simulink model "discrete_error_state_kalman"  (R2016a)
settings: Solver=VariableStepAuto  StartTime=0.0  StopTime=10.0  RelTol=1e-3
settings Model: Creator=mgreiff  LastModifiedBy=mgreiff
settings DataIOCC: LimitDataPoints=on
settings DebuggingCC: AllowSymbolicDim=off
settings ModelReferenceCC: PropagateSignalLabelsOutOfModel=off
settings GRTTargetCC: GeneratePreprocessorConditionals=Use local settings

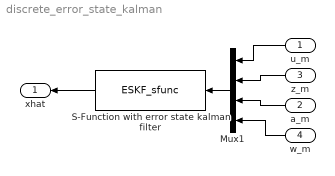
== system discrete_error_state_kalman ==
  u_m : Inport  PortDimensions=ESKFparam.nC
  a_m : Inport  Port=2  PortDimensions=3
  z_m : Inport  Port=3  PortDimensions=ESKFparam.nZ
  w_m : Inport  Port=4  PortDimensions=3
  Mux1 : Mux
  S-Function with error state kalman filter : S-Function  FunctionName=ESKF_sfunc  Parameters=ESKFparam  SFunctionDeploymentMode=off  EnableBusSupport=off
  xhat : Outport
  wires:
  u_m/1 -> Mux1/1
  z_m/1 -> Mux1/2
  S-Function with error state kalman filter/1 -> xhat/1
  Mux1/1 -> S-Function with error state kalman filter/1
  a_m/1 -> Mux1/3
  w_m/1 -> Mux1/4
